simulink model "Copy_3_of_L1AC_NAVION_Latest3"  (R2018a)
settings: Solver=ode4  StartTime=0.0  StopTime=30  FixedStep=Ts/10  RelTol=1e-3
values from neighbouring files (symbols this model uses):
  Am_LAT = A_LATERAL-B_LATERAL*K_LAT    [TEST_NAVION_LAT.m]
  B_LAT = [Bm_LAT Bum_LAT]    [TEST_NAVION_LAT.m]
  Bm_LAT = B_LATERAL    [TEST_NAVION_LAT.m]
  Bum_LAT = [ 0 -Bm_LAT(3,1) Bm_LAT(2,1) Bm_LAT(2,1) ;0 -Bm_LAT(3,1) Bm_LAT(2,1) -Bm_LAT(2,1)]'    [TEST_NAVION_LAT.m]
  DiscreteD_Lateral = c2d(D_Lateral ,Ts)    [TEST_NAVION_LAT.m]
  DiscretesistemaLateral = c2d(sistemaLateral,Ts)    [TEST_NAVION_LAT.m]
  INPUT_DISTURBANCE = 0    [MONTECARLO.m]    (also in run_control.m)
  K_const_LAT = 2.5*eye(2)    [TEST_NAVION_LAT.m]
  K_LAT = place(A_LATERAL,B_LATERAL,pole_TARGET_LAT)    [POLE_PLACEMENT.m]
  K_LONG = place (A_LONG , B_LONG , pole_TARGET_LONG)    [POLE_PLACEMENT.m]
  Kg_LAT = -(C_LAT*Am_LAT^-1*Bm_LAT)^-1    [TEST_NAVION_LAT.m]
  Ksp_LAT = -eye(size(Am_LAT))*0    [TEST_NAVION_LAT.m]
  omega0 = eye(2)    [TEST_NAVION_LAT.m]
  omega_true = eye(4)    [MONTECARLO.m]    (also in SETUP.m; run_control.m)
  OUTPUT_DISTURBANCE = 0    [MONTECARLO.m]    (also in run_control.m)
  PARAMETERS_AC = [g rho*8/8 c b S CL_0 CL_alpha CL_eq CL_de CD_0 AR e CY_beta CY_dr      Tmax Cl_beta Cl_p Cl_r Cl_da Cl_dr Cm_0 Cm_alpha Cm_eq Cm_de      Cn_beta  Cn_p Cn_r Cn_da Cn_dr m Ixx Iyy Izz]    [INIT.m]    (also in INIT_temp.m)
  sistemaLateral = ss(TF_eta2m,'minimal')    [TEST_NAVION_LAT.m]
  target_point = stato_trim_body    [SETUP.m]    (also in run_control.m)
  trim_input = stato(end-3:end)    [TRIM.m]
  Ts = 0.01    [MONTECARLO.m]    (also in run_control.m)
  Ts_delay = 1*Ts    [SETUP.m]    (also in run_control.m = 0.01)
  VARIANCE = diag( [ones( 12 , 1 )] )*1e-9    [MONTECARLO.m]    (also in run_control.m)
  x0 = stato_trim_body    [SETUP.m]    (also in TRIM.m = zeros( 16 , 1); run_control.m)
  x0hat_LAT = x0_new_LAT    [TEST_NAVION_LAT.m]
undefined symbols (not defined in the file or in its folder): Am, B, Bm, Bum, DiscIntNeverNeededParam, DiscreteD_Longitudinal, DiscretesistemaLongitudinal, K, Kg, Ksp, x0hat
libraries: visionstatistics x4, dspmtrx3 x2, dspinverses x2, simulink x2, commnoisgen2 x1
settings Model: Creator=Paolo  LastModifiedBy=Wolfrain
settings DebuggingCC: AlgebraicLoopMsg=error  ArtificialAlgebraicLoopMsg=error  BlockPriorityViolationMsg=error  MinStepSizeMsg=error  SimStateInterfaceChecksumMismatchMsg=error  LibraryContextMissingDiagnostic=warning
settings CodeAppCC: StateflowObjectComments=on

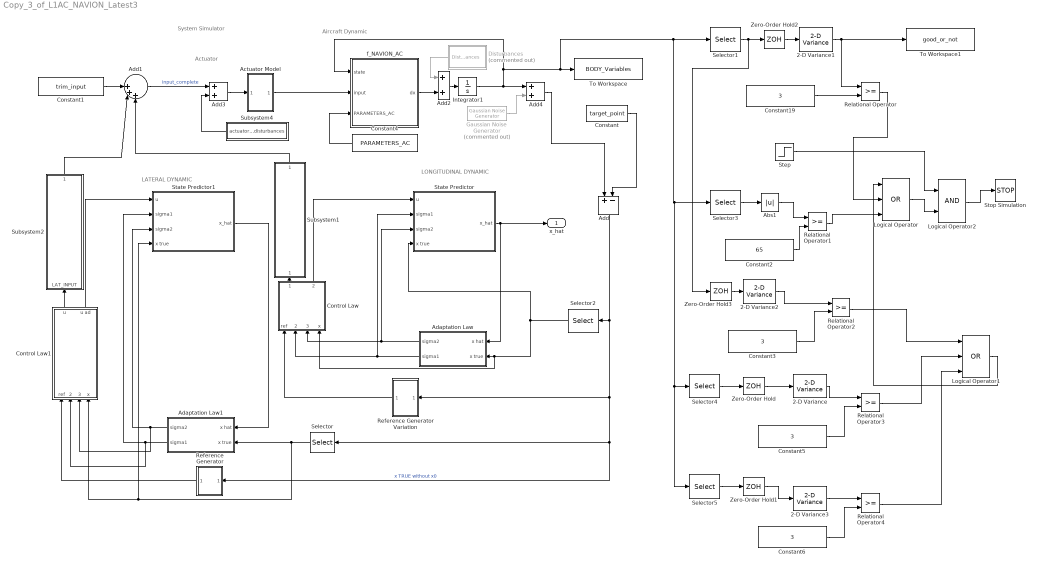
== system Copy_3_of_L1AC_NAVION_Latest3 ==
  note: Aircraft Dynamic
  note: Actuator
  note: LONGITUDINAL DYNAMIC
  note: LATERAL DYNAMIC
  note: System Simulator
  2-D Variance{,1..3} (4 alike) : visionstatistics/2-D Variance  run=on  reset_popup=None  directionMode=Entire input  dimension=1  treatSBRowAsCol=on  roiEnable=off  roiType=Rectangles  roiPortion=Entire ROI  roiOutput=Individual statistics for each ROI  roiFlag=off  prodOutputMode=Binary point scaling  prodOutputWordLength=32  prodOutputFracLength=0  roundingMode=Floor  overflowMode=off
      settings: SourceProductName=Computer Vision System Toolbox  SourceProductBaseCode=VP
  Abs1 : Abs
  Actuator Model : Subsystem
  Adaptation Law : Subsystem
  Adaptation Law1 : Subsystem
  Add : Sum  Inputs=+-
  Add1 : Sum  Inputs=||+++
  Add2 : Sum
  Add3 : Sum
  Add4 : Sum
  Constant : Constant  Value=target_point
  Constant1 : Constant  Value=trim_input
  Constant{3,5..6,19} (4 alike) : Constant  Value=3
  Constant2 : Constant  Value=65
  Constant4 : Constant  Value=PARAMETERS_AC
  Control Law : Subsystem
  Control Law1 : Subsystem
  Disturbances : Subsystem  Commented=on
  Gaussian Noise Generator : commnoisgen2/Gaussian Noise Generator  Commented=on  m=0  d=VARIANCE*1  s=41  Ts=Ts  frameBased=off  sampPerFrame=1  orient=off  outDataType=double
  Integrator1 : Integrator  InitialCondition=x0
  Logical Operator : Logic  Operator=OR  Inputs=3  AllPortsSameDT=off  OutDataTypeStr=boolean
  Logical Operator1 : Logic  Operator=OR  Inputs=3  AllPortsSameDT=off  OutDataTypeStr=boolean
  Logical Operator2 : Logic  AllPortsSameDT=off  OutDataTypeStr=boolean
  Reference Generator : Subsystem
  Reference Generator Variation : Subsystem
  Relational Operator{,1..4} (5 alike) : RelationalOperator  RndMeth=Nearest
  Selector : Selector  InputPortWidth=12  IndexOptions=Index vector (dialog)  Indices=[2 4 6 7]  OutputSizes=1
  Selector1 : Selector  InputPortWidth=12  IndexOptions=Index vector (dialog)  Indices=[1 2 3 4 5 6]  OutputSizes=1
  Selector2 : Selector  InputPortWidth=12  IndexOptions=Index vector (dialog)  Indices=[1 3 5 8]  OutputSizes=1
  Selector3 : Selector  InputPortWidth=12  IndexOptions=Index vector (dialog)  Indices=[9]  OutputSizes=1
  Selector4 : Selector  InputPortWidth=12  IndexOptions=Index vector (dialog)  Indices=[8]  OutputSizes=1
  Selector5 : Selector  InputPortWidth=12  IndexOptions=Index vector (dialog)  Indices=[7]  OutputSizes=1
  State Predictor : Subsystem
  State Predictor1 : Subsystem
  Step : Step  Time=20
  Stop Simulation : Stop
  Subsystem1 : Subsystem
  Subsystem2 : Subsystem
  Subsystem4 : Subsystem
  To Workspace : ToWorkspace  VariableName=BODY_Variables  SaveFormat=Timeseries  SampleTime=-1
  To Workspace1 : ToWorkspace  VariableName=good_or_not  SaveFormat=Timeseries  SampleTime=-1
  Zero-Order Hold{,1..3} (4 alike) : ZeroOrderHold  SampleTime=-1
  f_NAVION_AC : MATLAB Function  TreatAsAtomicUnit=on
  x_hat : Outport
  wires:
  Reference Generator Variation/1(Ref) -> Control Law/1(ref)
  Adaptation Law/2(sigma1) -> Control Law/2(sigma1), State Predictor/2(sigma1)
  Control Law/2(u_adaptive) -> State Predictor/1(u)
  Control Law/1(u_cmd_tot) -> Subsystem1/1(LONG_INPUT)
  Adaptation Law/1(sigma2) -> Control Law/3(sigma2), State Predictor/3(sigma2)
  State Predictor/1(x_hat) -> Adaptation Law/1(x hat), x_hat/1
  Add/1 -> Reference Generator/1(state), Selector/1, Reference Generator Variation/1(state), Selector2/1  "x TRUE without x0"
  Constant/1 -> Add/2
  Constant1/1 -> Add1/1
  Subsystem2/1(COMPATIBLE_INPUT_LAT) -> Add1/2
  Subsystem1/1(COMPATIBLE_INPUT_LONG) -> Add1/3
  Selector2/1 -> State Predictor/4(x true), Control Law/4(x), Adaptation Law/2(x true)
  Control Law1/1(u) -> Subsystem2/1(LAT_INPUT)
  Adaptation Law1/2(sigma1) -> Control Law1/2(sigma1), State Predictor1/2(sigma1)
  State Predictor1/1(x_hat) -> Adaptation Law1/1(x hat)
  Control Law1/2(u ad) -> State Predictor1/1(u)
  Selector/1 -> Control Law1/4(x), State Predictor1/4(x true), Adaptation Law1/2(x true)
  Reference Generator/1(Ref) -> Control Law1/1(ref)
  Adaptation Law1/1(sigma2) -> Control Law1/3(sigma2), State Predictor1/3(sigma2)
  Add1/1 -> Add3/1  "input_complete"
  Add3/1 -> Actuator Model/1(cmd)
  Subsystem4/1(actuators_ disturbances) -> Add3/2
  Disturbances/1(Disturbances) -> Add2/1
  Actuator Model/1(Fbk) -> f_NAVION_AC/2(input)
  Add2/1 -> Integrator1/1
  f_NAVION_AC/1(dx) -> Add2/2
  Constant4/1 -> f_NAVION_AC/3(PARAMETERS_AC)
  Add4/1 -> Add/1
  Gaussian Noise Generator/1 -> Add4/2
  2-D Variance1/1 -> To Workspace1/1, Relational Operator/1
  Constant19/1 -> Relational Operator/2
  Selector1/1 -> Zero-Order Hold3/1, Zero-Order Hold2/1
  Relational Operator/1 -> Logical Operator/2
  Relational Operator1/1 -> Logical Operator/3
  Selector3/1 -> Abs1/1
  Abs1/1 -> Relational Operator1/1
  Constant2/1 -> Relational Operator1/2
  2-D Variance2/1 -> Relational Operator2/1
  Constant3/1 -> Relational Operator2/2
  2-D Variance/1 -> Relational Operator3/1
  Constant5/1 -> Relational Operator3/2
  Constant6/1 -> Relational Operator4/2
  2-D Variance3/1 -> Relational Operator4/1
  Integrator1/1 -> Selector5/1, Selector4/1, Selector3/1, Selector1/1, To Workspace/1, f_NAVION_AC/1(state), Add4/1
  Relational Operator2/1 -> Logical Operator1/1
  Relational Operator3/1 -> Logical Operator1/2
  Relational Operator4/1 -> Logical Operator1/3
  Logical Operator1/1 -> Logical Operator/1
  Step/1 -> Logical Operator2/1
  Logical Operator/1 -> Logical Operator2/2
  Logical Operator2/1 -> Stop Simulation/1
  Zero-Order Hold/1 -> 2-D Variance/1
  Selector4/1 -> Zero-Order Hold/1
  Selector5/1 -> Zero-Order Hold1/1
  Zero-Order Hold1/1 -> 2-D Variance3/1
  Zero-Order Hold2/1 -> 2-D Variance1/1
  Zero-Order Hold3/1 -> 2-D Variance2/1

== system Copy_3_of_L1AC_NAVION_Latest3/Actuator Model ==
  cmd : Inport
  Constant2 : Constant  Value=omega_true
  Limiter and TF ACTUATOR1 : Subsystem
  Matrix Multiply : Product  Multiplication=Matrix(*)
  Quantizer : Quantizer  QuantizationInterval=1/(2^16-1)
  To Workspace1 : ToWorkspace  VariableName=INPUT_TO_ACTUATOR  SaveFormat=Timeseries  SampleTime=-1
  To Workspace2 : ToWorkspace  VariableName=ACTUATOR_TRUE  SaveFormat=Timeseries  SampleTime=-1
  Zero-Order Hold : ZeroOrderHold  SampleTime=Ts_delay
  Fbk : Outport
  wires:
  Limiter and TF ACTUATOR1/1(Out1) -> Matrix Multiply/2
  Constant2/1 -> Matrix Multiply/1
  Matrix Multiply/1 -> Fbk/1, To Workspace2/1
  Zero-Order Hold/1 -> Limiter and TF ACTUATOR1/1(In1)
  cmd/1 -> Quantizer/1, To Workspace1/1
  Quantizer/1 -> Zero-Order Hold/1

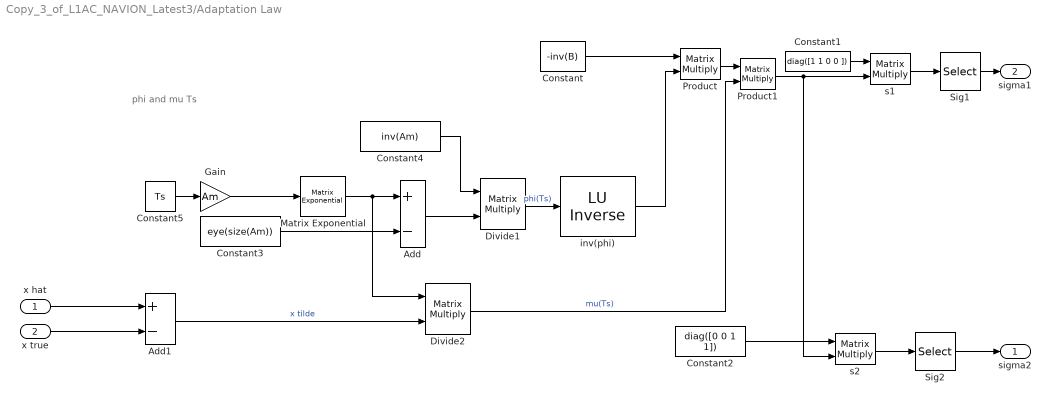
== system Copy_3_of_L1AC_NAVION_Latest3/Adaptation Law ==
  note: phi and mu Ts
  x hat : Inport
  x true : Inport  Port=2
  Add : Sum  Inputs=+-
  Add1 : Sum  Inputs=+-
  Constant : Constant  Value=-inv(B)
  Constant1 : Constant  Value=diag([1 1 0 0 ])
  Constant2 : Constant  Value=diag([0 0 1 1])
  Constant3 : Constant  Value=eye(size(Am))
  Constant4 : Constant  Value=inv(Am)
  Constant5 : Constant  Value=Ts
  Divide1 : Product  Inputs=**  Multiplication=Matrix(*)
  Divide2 : Product  Inputs=**  Multiplication=Matrix(*)
  Gain : Gain  Gain=Am
  Matrix Exponential : dspmtrx3/Matrix Exponential
      settings: SourceProductName=DSP System Toolbox  SourceProductBaseCode=DS
  Product : Product  Multiplication=Matrix(*)
  Product1 : Product  Multiplication=Matrix(*)
  Sig1 : Selector  InputPortWidth=4  IndexOptions=Index vector (dialog)  Indices=[1 2]  OutputSizes=1
  Sig2 : Selector  InputPortWidth=4  IndexOptions=Index vector (dialog)  Indices=[3 4]  OutputSizes=1
  inv(phi) : dspinverses/ LU Inverse
      settings: SourceProductName=DSP System Toolbox
  s1 : Product  Multiplication=Matrix(*)
  s2 : Product  Multiplication=Matrix(*)
  sigma2 : Outport
  sigma1 : Outport  Port=2
  wires:
  s2/1 -> Sig2/1
  Product/1 -> Product1/1
  Product1/1 -> s1/2, s2/2
  Constant/1 -> Product/1
  inv(phi)/1 -> Product/2
  Divide2/1 -> Product1/2  "mu(Ts)"
  Divide1/1 -> inv(phi)/1  "phi(Ts)"
  s1/1 -> Sig1/1
  Constant1/1 -> s1/1
  Constant2/1 -> s2/1
  Sig1/1 -> sigma1/1
  Sig2/1 -> sigma2/1
  Constant4/1 -> Divide1/1
  Constant5/1 -> Gain/1
  Matrix Exponential/1 -> Divide2/1, Add/1
  Add/1 -> Divide1/2
  x true/1 -> Add1/2
  Constant3/1 -> Add/2
  Add1/1 -> Divide2/2  "x tilde"
  x hat/1 -> Add1/1
  Gain/1 -> Matrix Exponential/1

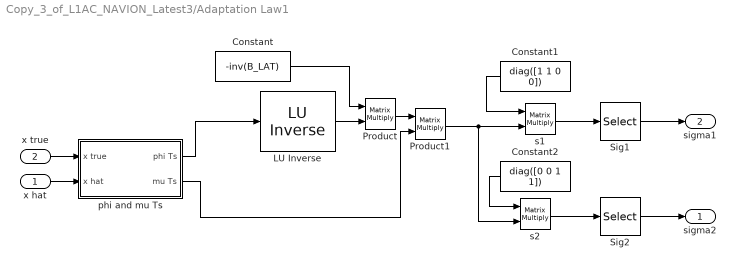
== system Copy_3_of_L1AC_NAVION_Latest3/Adaptation Law1 ==
  x hat : Inport
  x true : Inport  Port=2
  " LU Inverse" : dspinverses/ LU Inverse
      settings: SourceProductName=DSP System Toolbox
  Constant : Constant  Value=-inv(B_LAT)
  Constant1 : Constant  Value=diag([1 1 0 0])
  Constant2 : Constant  Value=diag([0 0 1 1])
  Product : Product  Multiplication=Matrix(*)
  Product1 : Product  Multiplication=Matrix(*)
  Sig1 : Selector  InputPortWidth=4  IndexOptions=Index vector (dialog)  Indices=[1 2]  OutputSizes=1
  Sig2 : Selector  InputPortWidth=4  IndexOptions=Index vector (dialog)  Indices=[3 4]  OutputSizes=1
  phi and mu Ts : Subsystem
  s1 : Product  Multiplication=Matrix(*)
  s2 : Product  Multiplication=Matrix(*)
  sigma2 : Outport
  sigma1 : Outport  Port=2
  wires:
  s2/1 -> Sig2/1
  Product/1 -> Product1/1
  Product1/1 -> s2/2, s1/2
  Constant/1 -> Product/1
  " LU Inverse"/1 -> Product/2
  phi and mu Ts/2(mu Ts) -> Product1/2
  phi and mu Ts/1(phi Ts) -> " LU Inverse"/1
  x hat/1 -> phi and mu Ts/2(x hat)
  x true/1 -> phi and mu Ts/1(x true)
  s1/1 -> Sig1/1
  Constant1/1 -> s1/1
  Constant2/1 -> s2/1
  Sig1/1 -> sigma1/1
  Sig2/1 -> sigma2/1

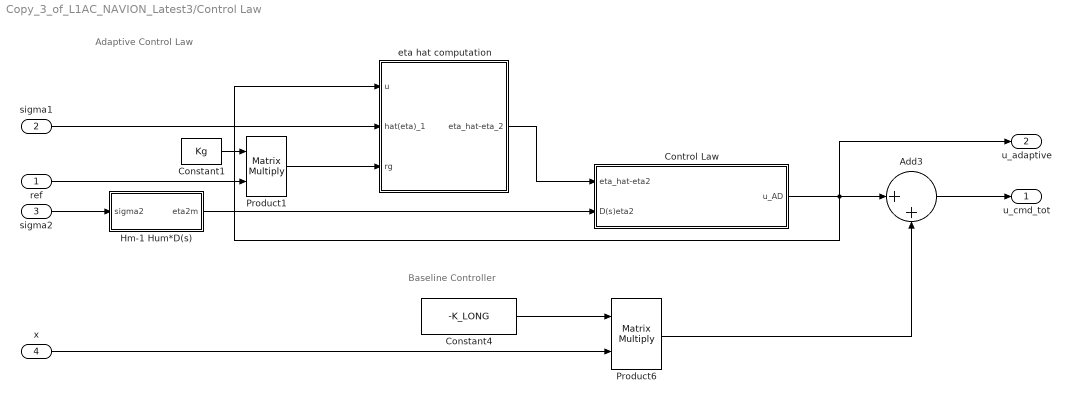
== system Copy_3_of_L1AC_NAVION_Latest3/Control Law ==
  note: Adaptive Control Law
  note: Baseline Controller
  ref : Inport
  sigma1 : Inport  Port=2
  sigma2 : Inport  Port=3
  x : Inport  Port=4
  Add3 : Sum  Inputs=|++
  Constant1 : Constant  Value=Kg
  Constant4 : Constant  Value=-K_LONG
  Control Law : Subsystem
  Hm-1 Hum*D(s) : Subsystem
  Product1 : Product  Multiplication=Matrix(*)  RndMeth=Zero
  Product6 : Product  Multiplication=Matrix(*)  RndMeth=Zero
  eta hat computation : Subsystem
  u_cmd_tot : Outport
  u_adaptive : Outport  Port=2
  wires:
  Add3/1 -> u_cmd_tot/1
  Product6/1 -> Add3/2
  Constant4/1 -> Product6/1
  x/1 -> Product6/2
  Control Law/1(u_AD) -> Add3/1, u_adaptive/1, eta hat computation/1(u)
  Hm-1 Hum*D(s)/1(eta2m) -> Control Law/2(D(s)eta2)
  Constant1/1 -> Product1/1
  Product1/1 -> eta hat computation/3(rg)
  ref/1 -> Product1/2
  sigma1/1 -> eta hat computation/2(hat(eta)_1)
  eta hat computation/1(eta_hat-eta_2) -> Control Law/1(eta_hat-eta2)
  sigma2/1 -> Hm-1 Hum*D(s)/1(sigma2)

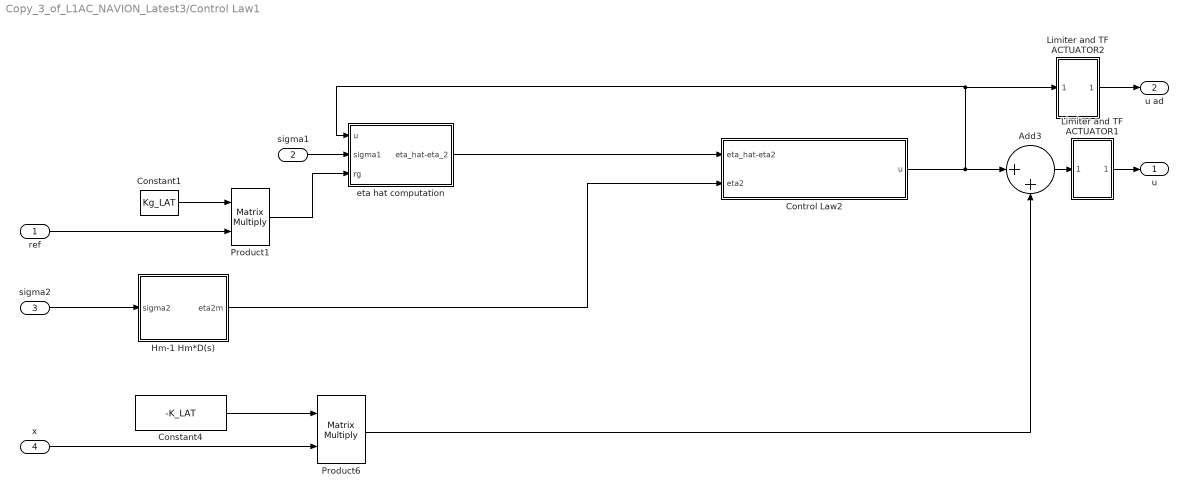
== system Copy_3_of_L1AC_NAVION_Latest3/Control Law1 ==
  ref : Inport
  sigma1 : Inport  Port=2
  sigma2 : Inport  Port=3
  x : Inport  Port=4
  Add3 : Sum  Inputs=|++
  Constant1 : Constant  Value=Kg_LAT
  Constant4 : Constant  Value=-K_LAT
  Control Law2 : Subsystem
  Hm-1 Hm*D(s) : Subsystem
  Limiter and TF ACTUATOR1 : Subsystem
  Limiter and TF ACTUATOR2 : Subsystem
  Product1 : Product  Multiplication=Matrix(*)  RndMeth=Zero
  Product6 : Product  Multiplication=Matrix(*)  RndMeth=Zero
  eta hat computation : Subsystem
  u : Outport
  u ad : Outport  Port=2
  wires:
  sigma2/1 -> Hm-1 Hm*D(s)/1(sigma2)
  eta hat computation/1(eta_hat-eta_2) -> Control Law2/1(eta_hat-eta2)
  sigma1/1 -> eta hat computation/2(sigma1)
  Control Law2/1(u) -> Add3/1, Limiter and TF ACTUATOR2/1(In1), eta hat computation/1(u)
  Hm-1 Hm*D(s)/1(eta2m) -> Control Law2/2(eta2)
  Product1/1 -> eta hat computation/3(rg)
  Add3/1 -> Limiter and TF ACTUATOR1/1(In1)
  Product6/1 -> Add3/2
  Constant4/1 -> Product6/1
  x/1 -> Product6/2
  Constant1/1 -> Product1/1
  ref/1 -> Product1/2
  Limiter and TF ACTUATOR1/1(Out1) -> u/1
  Limiter and TF ACTUATOR2/1(Out1) -> u ad/1

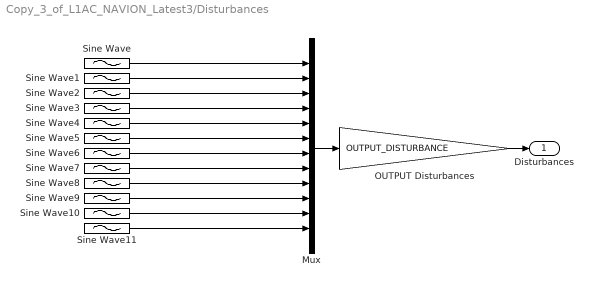
== system Copy_3_of_L1AC_NAVION_Latest3/Disturbances ==
  Mux : Mux  Inputs=12
  OUTPUT Disturbances : Gain  Gain=OUTPUT_DISTURBANCE
  Sine Wave : Sin  Amplitude=0.1  Frequency=3  SampleTime=0
  Sine Wave1 : Sin  Amplitude=0.2  Bias=0.1  Frequency=3  SampleTime=0
  Sine Wave10 : Sin  Amplitude=0.5  Frequency=3  SampleTime=0
  Sine Wave11 : Sin  Amplitude=0.8  Bias=2  Frequency=3  SampleTime=0
  Sine Wave2 : Sin  Amplitude=0.1  Frequency=0.5  SampleTime=0
  Sine Wave3 : Sin  Amplitude=0.1  SampleTime=0
  Sine Wave4 : Sin  Frequency=3  SampleTime=0
  Sine Wave5 : Sin  Amplitude=0.25  Frequency=3  SampleTime=0
  Sine Wave6 : Sin  Amplitude=0.2  Frequency=6  SampleTime=0
  Sine Wave7 : Sin  Amplitude=0.2  Frequency=3  SampleTime=0
  Sine Wave8 : Sin  Amplitude=0.5  Frequency=3  SampleTime=0
  Sine Wave9 : Sin  Amplitude=0.5  Frequency=3  SampleTime=0
  Disturbances : Outport
  wires:
  Mux/1 -> OUTPUT Disturbances/1
  Sine Wave/1 -> Mux/1
  Sine Wave1/1 -> Mux/2
  Sine Wave11/1 -> Mux/12
  OUTPUT Disturbances/1 -> Disturbances/1
  Sine Wave2/1 -> Mux/3
  Sine Wave3/1 -> Mux/4
  Sine Wave4/1 -> Mux/5
  Sine Wave5/1 -> Mux/6
  Sine Wave6/1 -> Mux/7
  Sine Wave7/1 -> Mux/8
  Sine Wave8/1 -> Mux/9
  Sine Wave9/1 -> Mux/10
  Sine Wave10/1 -> Mux/11

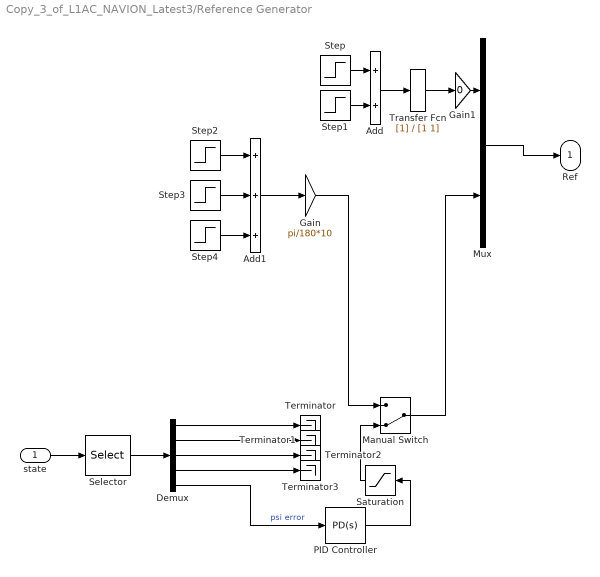
== system Copy_3_of_L1AC_NAVION_Latest3/Reference Generator ==
  state : Inport
  Add : Sum
  Add1 : Sum  Inputs=+++
  Demux : Demux  Outputs=5
  Gain : Gain  Gain=pi/180*10
  Gain1 : Gain  Gain=0
  Manual Switch : ManualSwitch  CurrentSetting=0
  Mux : Mux  Inputs=2
  PID Controller : simulink/Continuous/PID Controller  Controller=PD  TimeDomain=Continuous-time  SampleTime=-1  IntegratorMethod=Forward Euler  FilterMethod=Forward Euler  Form=Parallel  UseFilter=on  ControllerParametersSource=internal  P=-5  I=0  D=-5*0  N=20  InitialConditionSource=internal  InitialConditionForIntegrator=0  InitialConditionForFilter=0  ExternalReset=none  LimitOutput=on  UpperSaturationLimit=30/60  LowerSaturationLimit=-30/60  LinearizeAsGain=on  AntiWindupMode=back-calculation  Kb=1  TrackingMode=off  Kt=1  PParamMin=[]  PParamMax=[]  IParamMin=[]  IParamMax=[]  DParamMin=[]  DParamMax=[]  NParamMin=[]  NParamMax=[]  KbParamMin=[]  KbParamMax=[]  KtParamMin=[]  KtParamMax=[]  POutMin=[]  POutMax=[]  IOutMin=[]  IOutMax=[]  DOutMin=[]  DOutMax=[]  NOutMin=[]  NOutMax=[]  KbOutMin=[]  KbOutMax=[]  KtOutMin=[]  KtOutMax=[]  IntegratorOutMin=[]  IntegratorOutMax=[]  FilterOutMin=[]  FilterOutMax=[]  SumOutMin=[]  SumOutMax=[]  SumI1OutMin=[]  SumI1OutMax=[]  SumI2OutMin=[]  SumI2OutMax=[]  SumI3OutMin=[]  SumI3OutMax=[]  SumDOutMin=[]  SumDOutMax=[]  SaturationOutMin=[]  SaturationOutMax=[]  IntegratorContinuousStateAttributes=''  IntegratorStateMustResolveToSignalObject=off  IntegratorRTWStateStorageClass=Auto  FilterContinuousStateAttributes=''  FilterStateMustResolveToSignalObject=off  FilterRTWStateStorageClass=Auto  DifferentiatorICPrevScaledInput=0  DifferentiatorOutMin=[]  DifferentiatorOutMax=[]  FilterDiffOutCoefMin=[]  FilterDiffOutCoefMax=[]  SumDenOutMin=[]  SumDenOutMax=[]  SumNumOutMin=[]  SumNumOutMax=[]  ReciprocalOutMin=[]  ReciprocalOutMax=[]  DivideOutMin=[]  DivideOutMax=[]  TunerSelectOption=Transfer Function Based (PID Tuner App)
  Saturation : Saturate  UpperLimit=100  LowerLimit=-100
  Selector : Selector  InputPortWidth=12  IndexOptions=Index vector (dialog)  Indices=[2 4 6 7 9]  OutputSizes=1
  Step : Step  Time=2  After=4  SampleTime=0
  Step1 : Step  Time=20  After=-4  SampleTime=0
  Step2 : Step  Time=1.5  SampleTime=0
  Step3 : Step  Time=7.5+25  After=-2  SampleTime=0
  Step4 : Step  Time=15+25+25  After=+1  SampleTime=0
  Terminator{,1..3} (4 alike) : Terminator
  Transfer Fcn : TransferFcn  Denominator=[1 1]
  Ref : Outport
  wires:
  Step3/1 -> Add1/2
  Step4/1 -> Add1/3
  Mux/1 -> Ref/1
  Step2/1 -> Add1/1
  Step1/1 -> Add/2
  Step/1 -> Add/1
  Add/1 -> Transfer Fcn/1
  Gain1/1 -> Mux/1
  Transfer Fcn/1 -> Gain1/1
  Demux/2 -> Terminator1/1
  state/1 -> Selector/1
  Demux/3 -> Terminator2/1
  Demux/1 -> Terminator/1
  Saturation/1 -> Manual Switch/2
  Demux/5 -> PID Controller/1  "psi error"
  PID Controller/1 -> Saturation/1
  Add1/1 -> Gain/1
  Gain/1 -> Manual Switch/1
  Selector/1 -> Demux/1
  Demux/4 -> Terminator3/1
  Manual Switch/1 -> Mux/2

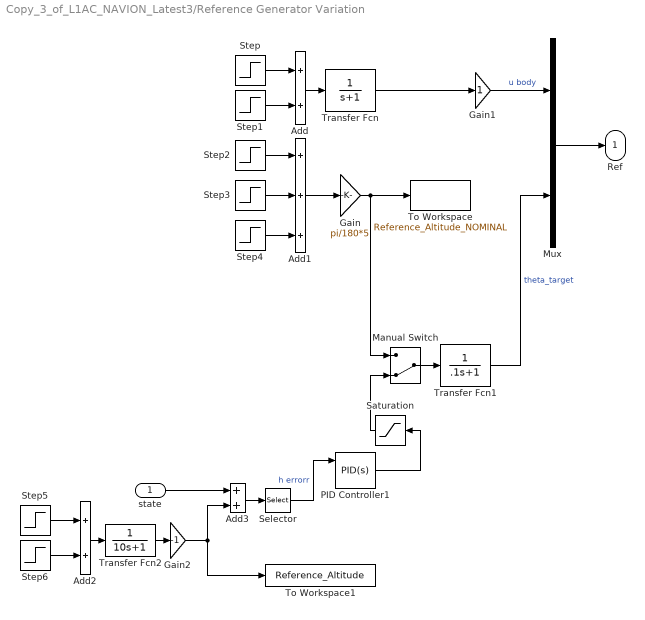
== system Copy_3_of_L1AC_NAVION_Latest3/Reference Generator Variation ==
  state : Inport
  Add : Sum
  Add1 : Sum  Inputs=+++
  Add2 : Sum
  Add3 : Sum
  Gain : Gain  Gain=pi/180*5
  Gain1 : Gain
  Gain2 : Gain  Gain=-1
  Manual Switch : ManualSwitch  CurrentSetting=0
  Mux : Mux  Inputs=2
  PID Controller1 : simulink/Continuous/PID Controller  Controller=PID  TimeDomain=Continuous-time  SampleTime=-1  IntegratorMethod=Forward Euler  FilterMethod=Forward Euler  Form=Parallel  UseFilter=on  ControllerParametersSource=internal  P=-.04/60*20  I=-0.004/60/2  D=0  N=60.8184531710771  InitialConditionSource=external  InitialConditionForIntegrator=0  InitialConditionForFilter=0  ExternalReset=none  LimitOutput=on  UpperSaturationLimit=10/60  LowerSaturationLimit=-10/60  LinearizeAsGain=on  AntiWindupMode=back-calculation  Kb=1  TrackingMode=off  Kt=1  PParamMin=[]  PParamMax=[]  IParamMin=[]  IParamMax=[]  DParamMin=[]  DParamMax=[]  NParamMin=[]  NParamMax=[]  KbParamMin=[]  KbParamMax=[]  KtParamMin=[]  KtParamMax=[]  POutMin=[]  POutMax=[]  IOutMin=[]  IOutMax=[]  DOutMin=[]  DOutMax=[]  NOutMin=[]  NOutMax=[]  KbOutMin=[]  KbOutMax=[]  KtOutMin=[]  KtOutMax=[]  IntegratorOutMin=[]  IntegratorOutMax=[]  FilterOutMin=[]  FilterOutMax=[]  SumOutMin=[]  SumOutMax=[]  SumI1OutMin=[]  SumI1OutMax=[]  SumI2OutMin=[]  SumI2OutMax=[]  SumI3OutMin=[]  SumI3OutMax=[]  SumDOutMin=[]  SumDOutMax=[]  SaturationOutMin=[]  SaturationOutMax=[]  IntegratorContinuousStateAttributes=''  IntegratorStateMustResolveToSignalObject=off  IntegratorRTWStateStorageClass=Auto  FilterContinuousStateAttributes=''  FilterStateMustResolveToSignalObject=off  FilterRTWStateStorageClass=Auto  DifferentiatorICPrevScaledInput=0  DifferentiatorOutMin=[]  DifferentiatorOutMax=[]  FilterDiffOutCoefMin=[]  FilterDiffOutCoefMax=[]  SumDenOutMin=[]  SumDenOutMax=[]  SumNumOutMin=[]  SumNumOutMax=[]  ReciprocalOutMin=[]  ReciprocalOutMax=[]  DivideOutMin=[]  DivideOutMax=[]  TunerSelectOption=Transfer Function Based (PID Tuner App)
  Saturation : Saturate  UpperLimit=100  LowerLimit=-100
  Selector : Selector  InputPortWidth=12  IndexOptions=Index vector (dialog)  Indices=[12]  OutputSizes=1
  Step : Step  Time=100  SampleTime=0
  Step1 : Step  Time=120  After=0  SampleTime=0
  Step2 : Step  Time=25  SampleTime=0
  Step3 : Step  Time=7.5+50  After=-2  SampleTime=0
  Step4 : Step  Time=15+50  After=+1  SampleTime=0
  Step5 : Step  Time=30  After=120  SampleTime=0
  Step6 : Step  Time=100  After=-50  SampleTime=0
  To Workspace : ToWorkspace  VariableName=Reference_Altitude_NOMINAL  SaveFormat=Timeseries  SampleTime=-1
  To Workspace1 : ToWorkspace  VariableName=Reference_Altitude  SaveFormat=Timeseries  SampleTime=-1
  Transfer Fcn : TransferFcn  Denominator=[1 1]
  Transfer Fcn1 : TransferFcn  Denominator=[.1 1]
  Transfer Fcn2 : TransferFcn  Denominator=[10 1]
  Ref : Outport
  wires:
  Step3/1 -> Add1/2
  Step4/1 -> Add1/3
  Mux/1 -> Ref/1
  Step2/1 -> Add1/1
  Step1/1 -> Add/2
  Step/1 -> Add/1
  Add/1 -> Transfer Fcn/1
  Gain1/1 -> Mux/1  "u body"
  Gain/1 -> To Workspace/1, Manual Switch/1
  Add1/1 -> Gain/1
  Transfer Fcn/1 -> Gain1/1
  Transfer Fcn1/1 -> Mux/2  "theta_target"
  Selector/1 -> PID Controller1/1  "h errorr"
  PID Controller1/1 -> Saturation/1
  Saturation/1 -> Manual Switch/2
  Manual Switch/1 -> Transfer Fcn1/1
  Add2/1 -> Transfer Fcn2/1
  state/1 -> Add3/1
  Step6/1 -> Add2/2
  Transfer Fcn2/1 -> Gain2/1
  Gain2/1 -> To Workspace1/1, Add3/2
  Step5/1 -> Add2/1
  Add3/1 -> Selector/1

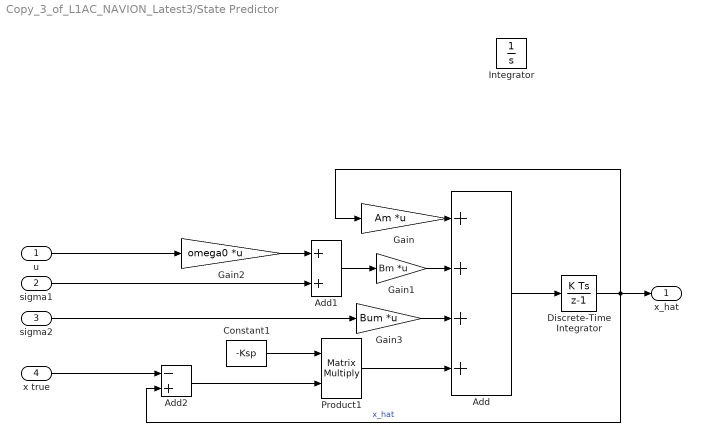
== system Copy_3_of_L1AC_NAVION_Latest3/State Predictor ==
  u : Inport
  sigma1 : Inport  Port=2
  sigma2 : Inport  Port=3
  x true : Inport  Port=4
  Add : Sum  Inputs=++++
  Add1 : Sum
  Add2 : Sum  Inputs=-+
  Constant1 : Constant  Value=-Ksp
  Discrete-Time Integrator : DiscreteIntegrator  InitialCondition=x0hat  SampleTime=-1  ICPrevOutput=DiscIntNeverNeededParam  ICPrevScaledInput=DiscIntNeverNeededParam
  Gain : Gain  Gain=Am  Multiplication=Matrix(K*u)
  Gain1 : Gain  Gain=Bm  Multiplication=Matrix(K*u)
  Gain2 : Gain  Gain=omega0  Multiplication=Matrix(K*u)
  Gain3 : Gain  Gain=Bum  Multiplication=Matrix(K*u)
  Integrator : Integrator  InitialCondition=x0hat
  Product1 : Product  Multiplication=Matrix(*)  RndMeth=Zero
  x_hat : Outport
  wires:
  Discrete-Time Integrator/1 -> x_hat/1, Add2/2, Gain/1  "x_hat"
  Add1/1 -> Gain1/1
  Gain3/1 -> Add/3
  Gain1/1 -> Add/2
  Product1/1 -> Add/4
  Gain/1 -> Add/1
  Gain2/1 -> Add1/1
  Add/1 -> Discrete-Time Integrator/1
  u/1 -> Gain2/1
  sigma1/1 -> Add1/2
  sigma2/1 -> Gain3/1
  x true/1 -> Add2/1
  Constant1/1 -> Product1/1
  Add2/1 -> Product1/2

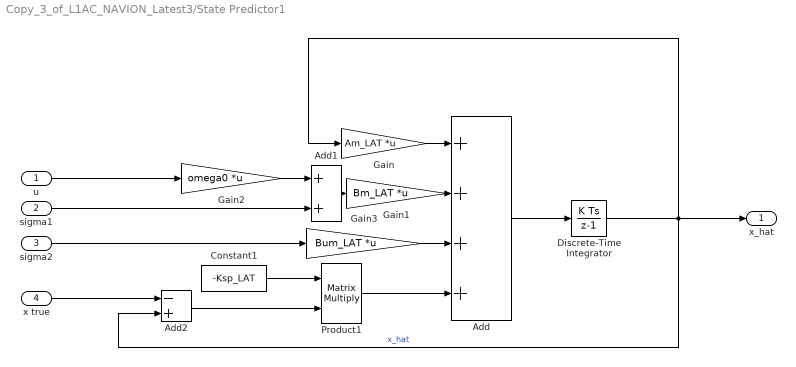
== system Copy_3_of_L1AC_NAVION_Latest3/State Predictor1 ==
  u : Inport
  sigma1 : Inport  Port=2
  sigma2 : Inport  Port=3
  x true : Inport  Port=4
  Add : Sum  Inputs=++++
  Add1 : Sum
  Add2 : Sum  Inputs=-+
  Constant1 : Constant  Value=-Ksp_LAT
  Discrete-Time Integrator : DiscreteIntegrator  InitialCondition=x0hat_LAT  SampleTime=-1  ICPrevOutput=DiscIntNeverNeededParam  ICPrevScaledInput=DiscIntNeverNeededParam
  Gain : Gain  Gain=Am_LAT  Multiplication=Matrix(K*u)
  Gain1 : Gain  Gain=Bm_LAT  Multiplication=Matrix(K*u)
  Gain2 : Gain  Gain=omega0  Multiplication=Matrix(K*u)
  Gain3 : Gain  Gain=Bum_LAT  Multiplication=Matrix(K*u)
  Product1 : Product  Multiplication=Matrix(*)  RndMeth=Zero
  x_hat : Outport
  wires:
  Discrete-Time Integrator/1 -> Add2/2, Gain/1, x_hat/1  "x_hat"
  Add1/1 -> Gain1/1
  Gain3/1 -> Add/3
  Gain1/1 -> Add/2
  Product1/1 -> Add/4
  Gain/1 -> Add/1
  Gain2/1 -> Add1/1
  Add/1 -> Discrete-Time Integrator/1
  u/1 -> Gain2/1
  sigma1/1 -> Add1/2
  sigma2/1 -> Gain3/1
  x true/1 -> Add2/1
  Constant1/1 -> Product1/1
  Add2/1 -> Product1/2

== system Copy_3_of_L1AC_NAVION_Latest3/Subsystem1 ==
  LONG_INPUT : Inport
  Constant16 : Constant  Value=0
  Demux1 : Demux  Outputs=2
  Mux2 : Mux
  COMPATIBLE_INPUT_LONG : Outport
  wires:
  Constant16/1 -> Mux2/2, Mux2/3
  Demux1/1 -> Mux2/1
  Demux1/2 -> Mux2/4
  Mux2/1 -> COMPATIBLE_INPUT_LONG/1
  LONG_INPUT/1 -> Demux1/1

== system Copy_3_of_L1AC_NAVION_Latest3/Subsystem2 ==
  LAT_INPUT : Inport
  Constant2 : Constant  Value=0
  Demux2 : Demux  Outputs=2
  Mux3 : Mux
  COMPATIBLE_INPUT_LAT : Outport
  wires:
  Constant2/1 -> Mux3/4, Mux3/1
  Mux3/1 -> COMPATIBLE_INPUT_LAT/1  "input lateral"
  Demux2/1 -> Mux3/2
  Demux2/2 -> Mux3/3
  LAT_INPUT/1 -> Demux2/1

== system Copy_3_of_L1AC_NAVION_Latest3/Subsystem4 ==
  INPUT Disturbances : Gain  Gain=INPUT_DISTURBANCE
  Mux : Mux
  Sine Wave : Sin  Amplitude=0.1  Frequency=3  SampleTime=0
  actuators_ disturbances : Outport
  wires:
  Mux/1 -> INPUT Disturbances/1
  Sine Wave/1 -> Mux/1, Mux/4, Mux/3, Mux/2
  INPUT Disturbances/1 -> actuators_ disturbances/1

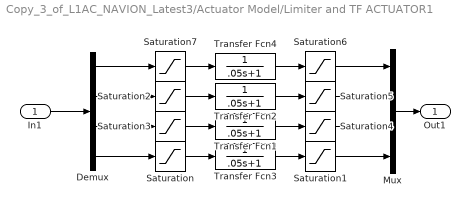
== system Copy_3_of_L1AC_NAVION_Latest3/Actuator Model/Limiter and TF ACTUATOR1 ==
  In1 : Inport
  Demux : Demux
  Mux : Mux
  Saturation : Saturate  UpperLimit=1  LowerLimit=0
  Saturation1 : Saturate  UpperLimit=1  LowerLimit=0
  Saturation{2..5} (4 alike) : Saturate  UpperLimit=0.3  LowerLimit=-0.3
  Saturation6 : Saturate  UpperLimit=20/60  LowerLimit=-20/60
  Saturation7 : Saturate  UpperLimit=20/60  LowerLimit=-20/60
  Transfer Fcn{1..4} (4 alike) : TransferFcn  Denominator=[.05 1]
  Out1 : Outport
  wires:
  Transfer Fcn2/1 -> Saturation5/1
  Transfer Fcn1/1 -> Saturation4/1
  Demux/3 -> Saturation3/1
  Saturation3/1 -> Transfer Fcn1/1
  Saturation2/1 -> Transfer Fcn2/1
  In1/1 -> Demux/1
  Transfer Fcn3/1 -> Saturation1/1
  Demux/2 -> Saturation2/1
  Mux/1 -> Out1/1
  Demux/4 -> Saturation/1
  Saturation/1 -> Transfer Fcn3/1
  Transfer Fcn4/1 -> Saturation6/1
  Demux/1 -> Saturation7/1
  Saturation1/1 -> Mux/4
  Saturation4/1 -> Mux/3
  Saturation5/1 -> Mux/2
  Saturation6/1 -> Mux/1
  Saturation7/1 -> Transfer Fcn4/1

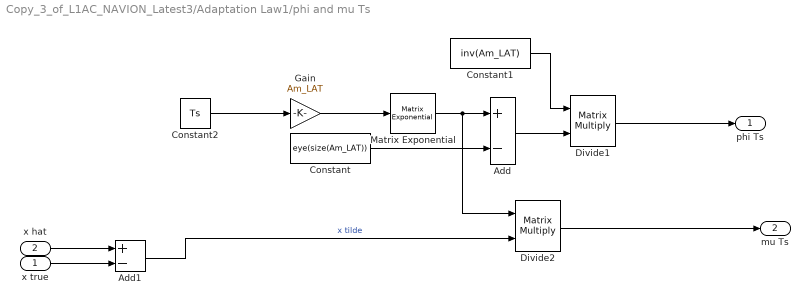
== system Copy_3_of_L1AC_NAVION_Latest3/Adaptation Law1/phi and mu Ts ==
  x true : Inport
  x hat : Inport  Port=2
  Add : Sum  Inputs=+-
  Add1 : Sum  Inputs=+-
  Constant : Constant  Value=eye(size(Am_LAT))
  Constant1 : Constant  Value=inv(Am_LAT)
  Constant2 : Constant  Value=Ts
  Divide1 : Product  Inputs=**  Multiplication=Matrix(*)
  Divide2 : Product  Inputs=**  Multiplication=Matrix(*)
  Gain : Gain  Gain=Am_LAT
  Matrix Exponential : dspmtrx3/Matrix Exponential
      settings: SourceProductName=DSP System Toolbox  SourceProductBaseCode=DS
  phi Ts : Outport
  mu Ts : Outport  Port=2
  wires:
  Gain/1 -> Matrix Exponential/1
  x hat/1 -> Add1/1
  Add1/1 -> Divide2/2  "x tilde"
  Divide1/1 -> phi Ts/1
  Constant/1 -> Add/2
  x true/1 -> Add1/2
  Add/1 -> Divide1/2
  Divide2/1 -> mu Ts/1
  Matrix Exponential/1 -> Divide2/1, Add/1
  Constant2/1 -> Gain/1
  Constant1/1 -> Divide1/1

== system Copy_3_of_L1AC_NAVION_Latest3/Control Law/Control Law ==
  note: D(s) eta\hat
  eta_hat-eta2 : Inport
  D(s)eta2 : Inport  Port=2
  Add2 : Sum
  Constant1 : Constant  Value=-K
  Discrete State-Space : DiscreteStateSpace  A=DiscreteD_Longitudinal.A  B=DiscreteD_Longitudinal.B  C=DiscreteD_Longitudinal.C  D=DiscreteD_Longitudinal.D  SampleTime=Ts
  Product1 : Product  Multiplication=Matrix(*)  RndMeth=Zero
  u_AD : Outport
  wires:
  eta_hat-eta2/1 -> Discrete State-Space/1
  Discrete State-Space/1 -> Add2/1  "D(s)(omega0*U_ad+\\hat\\eta1-rg)"
  Product1/1 -> u_AD/1
  D(s)eta2/1 -> Add2/2
  Constant1/1 -> Product1/1
  Add2/1 -> Product1/2

== system Copy_3_of_L1AC_NAVION_Latest3/Control Law/Hm-1 Hum*D(s) ==
  sigma2 : Inport
  Discrete State-Space : DiscreteStateSpace  A=DiscretesistemaLongitudinal.A  B=DiscretesistemaLongitudinal.B  C=DiscretesistemaLongitudinal.C  D=DiscretesistemaLongitudinal.D  SampleTime=Ts
  eta2m : Outport
  wires:
  sigma2/1 -> Discrete State-Space/1
  Discrete State-Space/1 -> eta2m/1

== system Copy_3_of_L1AC_NAVION_Latest3/Control Law/eta hat computation ==
  u : Inport
  hat(eta)_1 : Inport  Port=2
  rg : Inport  Port=3  PortDimensions=2
  Add : Sum  Inputs=++-
  Gain : Gain  Gain=omega0  Multiplication=Matrix(K*u)
  eta_hat-eta_2 : Outport
  wires:
  hat(eta)_1/1 -> Add/2
  Add/1 -> eta_hat-eta_2/1
  Gain/1 -> Add/1
  u/1 -> Gain/1
  rg/1 -> Add/3

== system Copy_3_of_L1AC_NAVION_Latest3/Control Law1/Control Law2 ==
  note: D(s)*eta
  eta_hat-eta2 : Inport
  eta2 : Inport  Port=2
  Add2 : Sum
  Constant1 : Constant  Value=-K_const_LAT
  Discrete State-Space : DiscreteStateSpace  A=DiscreteD_Lateral.A  B=DiscreteD_Lateral.B  C=DiscreteD_Lateral.C  D=DiscreteD_Lateral.D  SampleTime=Ts
  Product1 : Product  Multiplication=Matrix(*)  RndMeth=Zero
  u : Outport
  wires:
  eta_hat-eta2/1 -> Discrete State-Space/1
  Product1/1 -> u/1
  eta2/1 -> Add2/2
  Constant1/1 -> Product1/1
  Add2/1 -> Product1/2
  Discrete State-Space/1 -> Add2/1

== system Copy_3_of_L1AC_NAVION_Latest3/Control Law1/Hm-1 Hm*D(s) ==
  sigma2 : Inport
  Discrete State-Space : DiscreteStateSpace  A=DiscretesistemaLateral.A  B=DiscretesistemaLateral.B  C=DiscretesistemaLateral.C  D=DiscretesistemaLateral.D  SampleTime=Ts
  State-Space : StateSpace  A=sistemaLateral.A  B=sistemaLateral.B  C=sistemaLateral.C  D=sistemaLateral.D  InitialCondition=0
  eta2m : Outport
  wires:
  sigma2/1 -> Discrete State-Space/1
  Discrete State-Space/1 -> eta2m/1

== system Copy_3_of_L1AC_NAVION_Latest3/Control Law1/Limiter and TF ACTUATOR1 ==
  In1 : Inport
  Demux : Demux  Outputs=2
  Mux : Mux  Inputs=2
  Saturation2 : Saturate  UpperLimit=0.3  LowerLimit=-0.3
  Saturation3 : Saturate  UpperLimit=0.3  LowerLimit=-0.3
  Transfer Fcn1 : TransferFcn  Denominator=[0.05 1]
  Transfer Fcn2 : TransferFcn  Denominator=[0.5 1]
  Out1 : Outport
  wires:
  Demux/2 -> Saturation3/1
  Saturation3/1 -> Transfer Fcn1/1
  Saturation2/1 -> Transfer Fcn2/1
  In1/1 -> Demux/1
  Mux/1 -> Out1/1
  Transfer Fcn1/1 -> Mux/2
  Transfer Fcn2/1 -> Mux/1
  Demux/1 -> Saturation2/1

== system Copy_3_of_L1AC_NAVION_Latest3/Control Law1/Limiter and TF ACTUATOR2 ==
  In1 : Inport
  Demux : Demux  Outputs=2
  Mux : Mux  Inputs=2
  Saturation2 : Saturate  UpperLimit=0.3  LowerLimit=-0.3
  Saturation3 : Saturate  UpperLimit=0.3  LowerLimit=-0.3
  Transfer Fcn1 : TransferFcn  Denominator=[0.05 2]
  Transfer Fcn2 : TransferFcn  Denominator=[0.05 2]
  Out1 : Outport
  wires:
  Demux/1 -> Saturation2/1
  Transfer Fcn2/1 -> Mux/1
  Transfer Fcn1/1 -> Mux/2
  Mux/1 -> Out1/1
  In1/1 -> Demux/1
  Saturation2/1 -> Transfer Fcn2/1
  Saturation3/1 -> Transfer Fcn1/1
  Demux/2 -> Saturation3/1

== system Copy_3_of_L1AC_NAVION_Latest3/Control Law1/eta hat computation ==
  u : Inport
  sigma1 : Inport  Port=2
  rg : Inport  Port=3  PortDimensions=2
  Add : Sum  Inputs=++-
  Gain : Gain  Gain=omega0  Multiplication=Matrix(K*u)
  eta_hat-eta_2 : Outport
  wires:
  sigma1/1 -> Add/2
  Add/1 -> eta_hat-eta_2/1
  Gain/1 -> Add/1
  u/1 -> Gain/1
  rg/1 -> Add/3

== matlab function Copy_3_of_L1AC_NAVION_Latest3/f_NAVION_AC ==
  data: state input; dx output; input input; PARAMETERS_AC input
function dx = f_NAVION_SIMULINK(state,input,PARAMETERS_AC)
dx = zeros(12,1);
u = state(1);
v = state(2);
w = state(3);
p = state(4);
q = state(5);
r = state(6);
phi = state(7);
theta = state(8);
psi = state(9);
xg = state(10);
yg = state(11);
h = state(12);

de = input(1);
da = input(2);
dr = input(3);
dt = input(4);
%% Parameters AR = 6.04 e = 0.7 to implement into the setup
% global  g rho c b S CL_0 CL_alpha CL_eq CL_de CD_0 AR e CY_beta CY_dr ...
%         Tmax Cl_beta Cl_p Cl_r Cl_da Cl_dr Cm_0 Cm_alpha Cm_eq Cm_de ...
%         Cn_beta  Cn_p Cn_r Cn_da Cn_dr m Ixx Iyy Izz

g = PARAMETERS_AC(1);
rho = PARAMETERS_AC(2);
c = PARAMETERS_AC(3);
b = PARAMETERS_AC(4);
S = PARAMETERS_AC(5);
CL_0 = PARAMETERS_AC(6);
CL_alpha = PARAMETERS_AC(7);
CL_eq = PARAMETERS_AC(8);
CL_de = PARAMETERS_AC(9);
CD_0 = PARAMETERS_AC(10); 
AR = PARAMETERS_AC(11);
e = PARAMETERS_AC(12);
CY_beta = PARAMETERS_AC(13);
CY_dr = PARAMETERS_AC(14);
Tmax = PARAMETERS_AC(15);
Cl_beta = PARAMETERS_AC(16);
Cl_p = PARAMETERS_AC(17);
Cl_r = PARAMETERS_AC(18);
Cl_da = PARAMETERS_AC(19);
Cl_dr = PARAMETERS_AC(20);
Cm_0 = PARAMETERS_AC(21);
Cm_alpha = PARAMETERS_AC(22);
Cm_eq = PARAMETERS_AC(23);
Cm_de = PARAMETERS_AC(24);
Cn_beta = PARAMETERS_AC(25);
Cn_p = PARAMETERS_AC(26);
Cn_r = PARAMETERS_AC(27);
Cn_da = PARAMETERS_AC(28);
Cn_dr = PARAMETERS_AC(29);
m = PARAMETERS_AC(30);
Ixx = PARAMETERS_AC(31);
Iyy = PARAMETERS_AC(32);
Izz = PARAMETERS_AC(33);

%% From body to wind for forces and moments
V = sqrt(u^2+v^2+w^2);
alpha = atan(w/u);
beta = asin(v/V);
%% CL CD and CY construction
CL = CL_0+CL_alpha*alpha+CL_eq*(c/(2*V))*q+CL_de*de;
% alphamax = 15*pi/180;

% if alpha>alphamax
%     CL=CL_0+CL_alpha*alphamax+CL_eq*(c/(2*V))*q+CL_de*de;
%     CL=0;
% end

CD = CD_0 + (CL^2)/(pi*AR*e);
CY = CY_beta *beta +CY_dr *dr;
%% Forces
Lift = 1/2*rho *V^2*S*CL;
Drag = 1/2*rho *V^2*S*CD;
Side_Force = 1/2*rho *V^2*S*CY;
Thrust = dt*Tmax;
delta_engine = 0;
X_Thrust = Thrust * cos(delta_engine);
Z_Thrust= Thrust * sin(delta_engine);
Y_Thrust= 0;
%% Cl Cp Cn
Cl = Cl_beta*beta+Cl_p*(b/(2*V))*p+Cl_r *(b/(2*V))*r + Cl_da*da+Cl_dr*dr;
Cm = Cm_0+Cm_alpha*alpha+Cm_eq*(c/(2*V))*q+Cm_de*de; 
Cn = Cn_beta*beta + Cn_p *(b/(2*V))*p +Cn_r * (b/(2*V))*r + Cn_da*da+Cn_dr*dr;
%% Moments
ROLL_MOMENT = 1/2*rho*S*b*Cl*V^2;
PITCH_MOMENT = 1/2*rho*S*c*Cm*V^2;
YAW_MOMENT = 1/2*rho*S*b*Cn*V^2;

u_dot = (X_Thrust-g*m*sin(theta)-Drag*cos(alpha)+Lift*sin(alpha))/m + r*V*sin(beta)-q*V*sin(alpha)*cos(beta);
v_dot = (Y_Thrust+g*m*sin(phi)*cos(theta)+Side_Force)/m + p*V*sin(alpha)*cos(beta)-r*V*cos(alpha)*cos(beta);
w_dot = (Z_Thrust+g*m*cos(phi)*cos(theta)-Drag*sin(alpha)-Lift*cos(alpha))/m + q*V*cos(alpha)*cos(beta)-p*V*sin(beta);

p_dot = (ROLL_MOMENT  + (Iyy-Izz) *q*r)/Ixx;
q_dot = (PITCH_MOMENT + (Ixx-Izz) *p*r)/Iyy;
r_dot = (YAW_MOMENT+(Ixx-Iyy)*p*q)/Izz;

phi_dot = p+q*sin(phi)*tan(theta)+r*cos(phi)*tan(theta);
theta_dot = q*cos(phi)-r*sin(phi);
psi_dot = q*sin(phi)*sec(theta) + r*cos(phi)*sec(theta);

% xg_dot = u*cos(psi)*cos(theta)+v*(cos(psi)*sin(theta)*sin(phi)-sin(psi)*cos(phi))+w*(cos(psi)*sin(theta)*cos(phi)+sin(psi)*sin(phi));
% yg_dot = u*sin(psi)*cos(theta)+v*(sin(psi)*sin(theta)*sin(phi)+cos(psi)*cos(phi))+w*(sin(psi)*sin(theta)*cos(phi)-cos(psi)*sin(phi));
% h_dot  = u*sin(theta)-v*cos(theta)*sin(phi)-w*cos(theta)*cos(phi);

xg_dot = u*cos(psi)*cos(theta)+v*(cos(psi)*sin(theta)*sin(phi)-sin(psi)*cos(phi))+w*(cos(psi)*sin(theta)*cos(phi)+sin(psi)*sin(phi));
yg_dot = u*sin(psi)*cos(theta)+v*(sin(psi)*sin(theta)*sin(phi)+cos(psi)*cos(phi))+w*(sin(psi)*sin(theta)*cos(phi)-cos(psi)*sin(phi));
h_dot  = u*sin(theta)-v*cos(theta)*sin(phi)-w*cos(theta)*cos(phi);

dx = [u_dot v_dot w_dot p_dot q_dot r_dot phi_dot theta_dot psi_dot xg_dot yg_dot h_dot]';

end
